simulink model "POINTING_2"  (R2022b)
settings: Solver=VariableStepAuto  StartTime=0.0  StopTime=36000  RelTol=1e-3
values from neighbouring files (symbols this model uses):
  A0 = angle2dcm(E1+0.7,E2+0.4,E3-1)    [Pointing_tuning.m]
  K_cz = sat.I/sat.I(3)*1e-4    [Pointing_tuning.m]    (also in fitnessfcn.m = X(4:6))
  K_w = 1e-2    (= 0.01)    [Pointing_tuning.m]    (also in fitnessfcn.m = X(7))
  n = sqrt(settings.mu/settings.a^3)    [Pointing_tuning.m]    (also in control_tuning.m)
undefined symbols (not defined in the file or in its folder): environment, r0, sat, settings, v0
libraries: matrix_library x7, vrlib x4, cstblocks x1
settings Model: Creator=brent  LastModifiedBy=brent

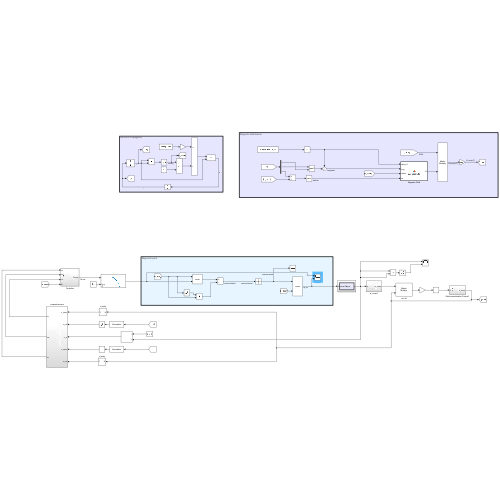
[thumbnail: Simulink's stored preview of the top-level diagram]
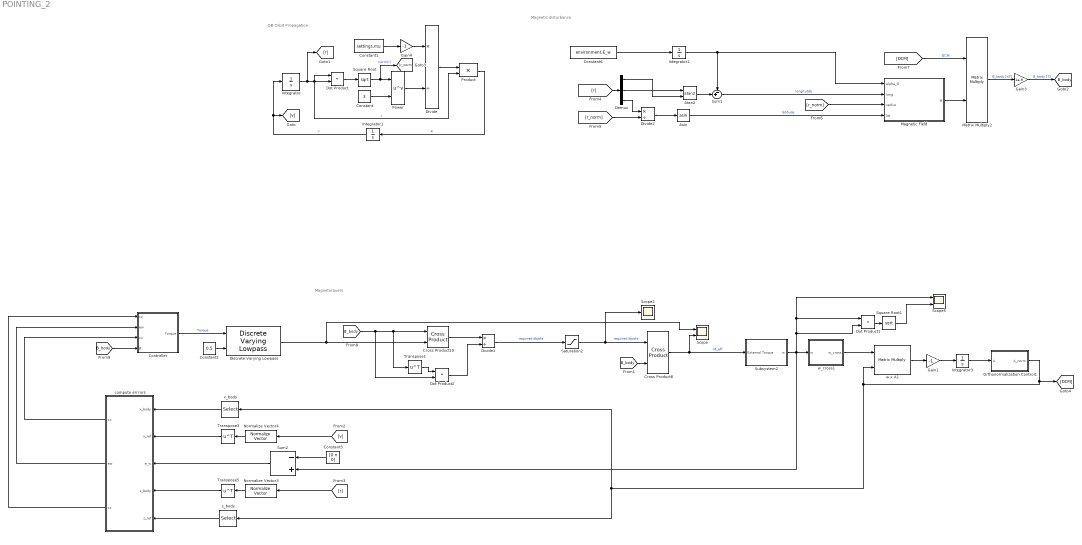
== system POINTING_2 ==
  note: Magnetic disturbance
  note: OB Orbit Propagation
  note: Magnetorquers
  " w x A1" : Product  Multiplication=Matrix(*)
  Asin : Trigonometry  Operator=asin
  Atan2 : Trigonometry  Operator=atan2
  Constant : Constant  Value=3
  Constant1 : Constant  Value=settings.mu
  Constant2 : Constant  Value=0.5
  Constant3 : Constant  Value=[0 n 0]
  Constant6 : Constant  Value=environment.E_w
  Controller : Subsystem
  Cross Product10 : matrix_library/Cross Product
  Cross Product8 : matrix_library/Cross Product
  Demux : Demux  Outputs=3
  Discrete Varying Lowpass : cstblocks/Linear Parameter Varying/Discrete Varying Lowpass  N=4  w0=0  Ts=1
  Divide : Product  Inputs=*/
  Divide1 : Product  Inputs=*/  RndMeth=Zero  SaturateOnIntegerOverflow=on
  Divide2 : Product  Inputs=*/
  Dot Product : DotProduct  OutDataTypeStr=Inherit: Inherit via internal rule
  Dot Product1 : DotProduct  OutDataTypeStr=Inherit: Inherit via internal rule
  Dot Product2 : DotProduct  OutDataTypeStr=Inherit: Inherit via internal rule
  Gain1 : Gain  Gain=-1
  Gain3 : Gain  Gain=1e-9
  Gain4 : Gain  Gain=-1
  Integrator : Integrator  InitialCondition=r0
  Integrator1 : Integrator  InitialCondition=v0
  Integrator2 : Integrator  InitialCondition=environment.theta_G0
  Integrator3 : Integrator  InitialCondition=A0
  Magnetic Field : MATLAB Function  TreatAsAtomicUnit=on
  Matrix Multiply2 : Product  Multiplication=Matrix(*)
  Normalize Vector3 : vrlib/Utilities/Normalize Vector  maxzero=0
  Normalize Vector4 : vrlib/Utilities/Normalize Vector  maxzero=0
  Orthonormalization Control1 : Subsystem
  Power : Math  Operator=pow
  Product : Product
  Saturation2 : Saturate  UpperLimit=120  LowerLimit=-120
  Scope : Scope  NumInputPorts=2
  Scope2 : Scope
  Scope5 : Scope  NumInputPorts=2
  Square Root : Sqrt
  Square Root1 : Sqrt
  Subsystem2 : Subsystem
  Sum1 : Sum  Inputs=-+|
  Sum2 : Sum  Inputs=-+
  Transpose1 : Math  Operator=transpose
  Transpose3 : Math  Operator=transpose
  Transpose5 : Math  Operator=transpose
  compute errrors : Subsystem
  w_cross1 : Subsystem
  x_body : Selector  NumberOfDimensions=2  InputPortWidth=3  IndexOptions=Index vector (dialog),Index vector (dialog)  Indices=[1],[1 2 3]  OutputSizes=1,1
  z_body : Selector  NumberOfDimensions=2  InputPortWidth=3  IndexOptions=Index vector (dialog),Index vector (dialog)  Indices=[3],[1 2 3]  OutputSizes=1,1
  tag scope: B_body=global
  wires:
  Divide2/1 -> Asin/1
  Constant6/1 -> Integrator2/1
  [DCM] -> Matrix Multiply2/1  "DCM"
  Demux/3 -> Divide2/1
  Matrix Multiply2/1 -> Gain3/1  "B_body [nT]"
  Demux/2 -> Atan2/1
  [r] -> Demux/1
  [r_norm] -> Magnetic Field/3(radius)
  Gain3/1 -> [B_body]  "B_body [T]"
  Demux/1 -> Atan2/2
  Integrator2/1 -> Sum1/1, Magnetic Field/1(alpha_G)
  Asin/1 -> Magnetic Field/4(lat)  "latitude"
  Atan2/1 -> Sum1/2
  Constant/1 -> Power/2
  Product/1 -> Integrator1/1  "a"
  Integrator/1 -> [r], Product/2, Dot Product/2, Dot Product/1  "r"
  Integrator1/1 -> [v], Integrator/1  "v"
  Dot Product/1 -> Square Root/1
  Magnetic Field/1(B) -> Matrix Multiply2/2
  Sum1/1 -> Magnetic Field/2(long)  "longitutde"
  Constant1/1 -> Gain4/1
  [r_norm] -> Divide2/2
  Power/1 -> Divide/2
  Gain4/1 -> Divide/1
  Square Root/1 -> [r_norm], Power/1  "norm(r)"
  Divide/1 -> Product/1
  Square Root1/1 -> Scope5/2
  Subsystem2/1(w) -> Sum2/2, w_cross1/1(w), Dot Product1/1, Scope5/1, Dot Product1/2
  Orthonormalization Control1/1(A_norm) -> [DCM], x_body/1, z_body/1, " w x A1"/2
  " w x A1"/1 -> Gain1/1
  w_cross1/1(w_cross) -> " w x A1"/1
  Integrator3/1 -> Orthonormalization Control1/1(A)
  Dot Product1/1 -> Square Root1/1
  Gain1/1 -> Integrator3/1
  [B_body] -> Transpose1/1, Cross Product10/1, Dot Product2/2
  Transpose1/1 -> Dot Product2/1
  Dot Product2/1 -> Divide1/2
  Cross Product10/1 -> Divide1/1
  Divide1/1 -> Saturation2/1  "required dipole"
  [B_body] -> Cross Product8/2
  Cross Product8/1 -> Scope/2, Subsystem2/1(External Torque)  "M_eff"
  Saturation2/1 -> Cross Product8/1, Scope2/1  "required dipole"
  Controller/1(Torque) -> Discrete Varying Lowpass/1  "Torque"
  Constant3/1 -> Sum2/1
  Discrete Varying Lowpass/1 -> Scope/1, Cross Product10/2
  Constant2/1 -> Discrete Varying Lowpass/2
  Normalize Vector4/1 -> Transpose3/1
  [r] -> Normalize Vector3/1
  [v] -> Normalize Vector4/1
  Normalize Vector3/1 -> Transpose5/1
  x_body/1 -> compute errrors/1(x_body)
  Transpose3/1 -> compute errrors/2(x_ref)
  Sum2/1 -> compute errrors/3(e_w)
  Transpose5/1 -> compute errrors/4(z_body)
  z_body/1 -> compute errrors/5(z_ref)
  compute errrors/1(cx) -> Controller/3(cx)
  compute errrors/2(ew) -> Controller/2(ew)
  compute errrors/3(cz) -> Controller/1(cz)
  [B_body] -> Controller/4(B)

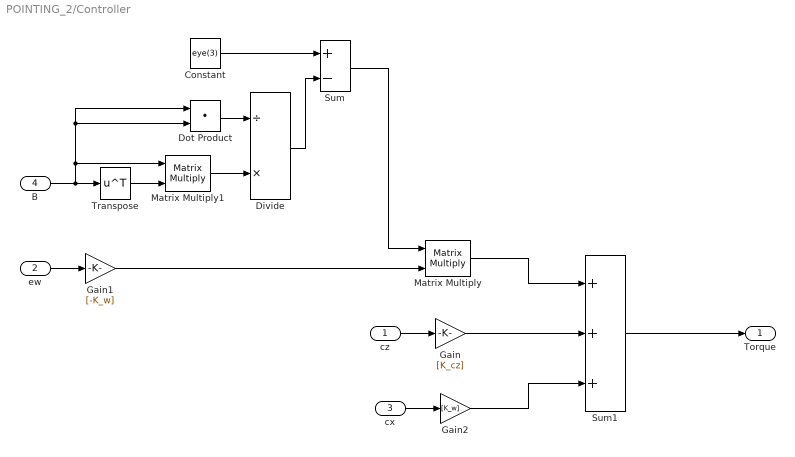
== system POINTING_2/Controller ==
  cz : Inport
  ew : Inport  Port=2
  cx : Inport  Port=3
  B : Inport  Port=4
  Constant : Constant  Value=eye(3)
  Divide : Product  Inputs=/*
  Dot Product : DotProduct  OutDataTypeStr=Inherit: Inherit via internal rule
  Gain : Gain  Gain=[K_cz]
  Gain1 : Gain  Gain=[-K_w]
  Gain2 : Gain  Gain=[K_w]
  Matrix Multiply : Product  Multiplication=Matrix(*)
  Matrix Multiply1 : Product  Multiplication=Matrix(*)
  Sum : Sum  Inputs=+-
  Sum1 : Sum  Inputs=+++
  Transpose : Math  Operator=transpose
  Torque : Outport
  wires:
  cz/1 -> Gain/1
  ew/1 -> Gain1/1
  cx/1 -> Gain2/1
  Gain1/1 -> Matrix Multiply/2
  Constant/1 -> Sum/1
  B/1 -> Dot Product/2, Dot Product/1, Matrix Multiply1/1, Transpose/1
  Transpose/1 -> Matrix Multiply1/2
  Matrix Multiply1/1 -> Divide/2
  Dot Product/1 -> Divide/1
  Divide/1 -> Sum/2
  Sum/1 -> Matrix Multiply/1
  Gain/1 -> Sum1/2
  Matrix Multiply/1 -> Sum1/1
  Gain2/1 -> Sum1/3
  Sum1/1 -> Torque/1

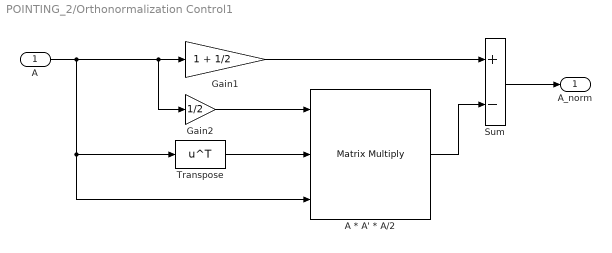
== system POINTING_2/Orthonormalization Control1 ==
  A : Inport
  " A * A' * A/2" : Product  Inputs=3  Multiplication=Matrix(*)
  Gain1 : Gain  Gain=1 + 1/2
  Gain2 : Gain  Gain=1/2
  Sum : Sum  Inputs=+-
  Transpose : Math  Operator=transpose
  A_norm : Outport
  wires:
  A/1 -> Transpose/1, " A * A' * A/2"/3, Gain1/1, Gain2/1
  Gain1/1 -> Sum/1
  " A * A' * A/2"/1 -> Sum/2
  Sum/1 -> A_norm/1
  Gain2/1 -> " A * A' * A/2"/1
  Transpose/1 -> " A * A' * A/2"/2

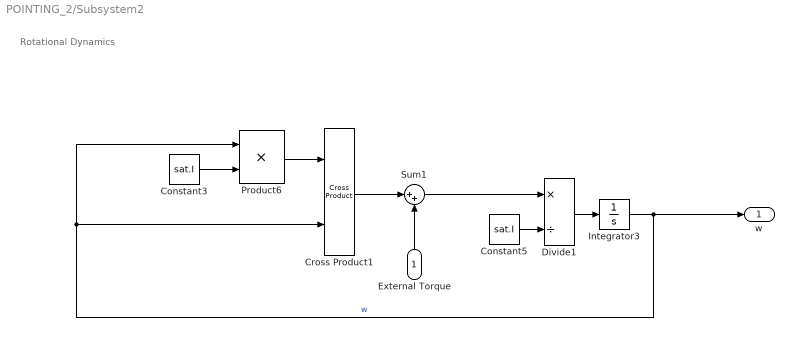
== system POINTING_2/Subsystem2 ==
  note: Rotational Dynamics
  External Torque : Inport
  Constant3 : Constant  Value=sat.I
  Constant5 : Constant  Value=sat.I
  Cross Product1 : matrix_library/Cross Product
  Divide1 : Product  Inputs=*/
  Integrator3 : Integrator  InitialCondition=settings.w0
  Product6 : Product
  Sum1 : Sum  Inputs=|++
  w : Outport
  wires:
  Constant5/1 -> Divide1/2
  Sum1/1 -> Divide1/1
  External Torque/1 -> Sum1/2
  Integrator3/1 -> w/1, Cross Product1/2, Product6/1  "w"
  Divide1/1 -> Integrator3/1
  Cross Product1/1 -> Sum1/1
  Constant3/1 -> Product6/2
  Product6/1 -> Cross Product1/1

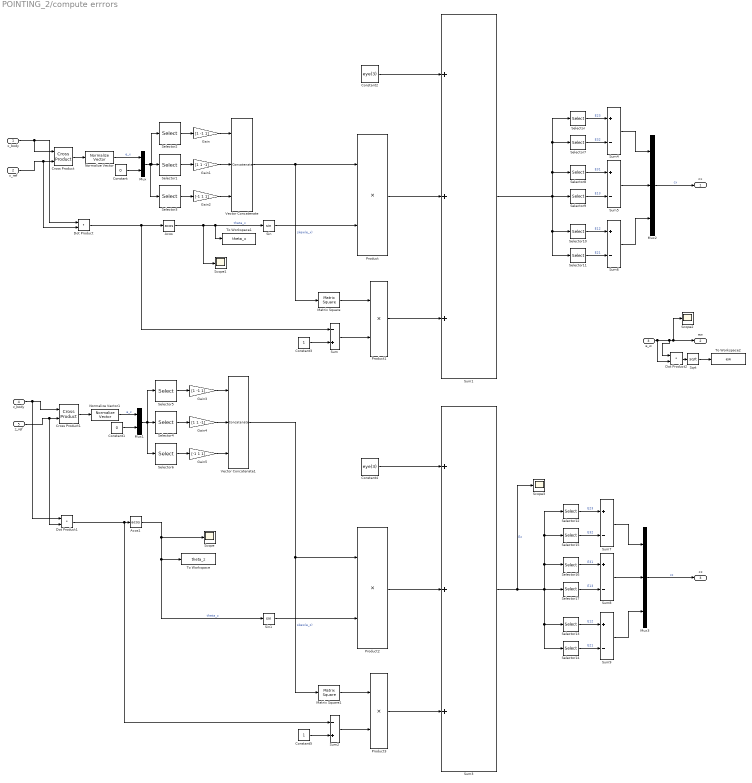
== system POINTING_2/compute errrors ==
  x_body : Inport
  x_ref : Inport  Port=2
  e_w : Inport  Port=3
  z_body : Inport  Port=4
  z_ref : Inport  Port=5
  Acos : Trigonometry  Operator=acos
  Acos1 : Trigonometry  Operator=acos
  Constant : Constant  Value=0
  Constant1 : Constant  Value=0
  Constant2 : Constant  Value=eye(3)
  Constant3 : Constant
  Constant4 : Constant  Value=eye(3)
  Constant5 : Constant
  Cross Product : matrix_library/Cross Product
  Cross Product1 : matrix_library/Cross Product
  Dot Product : DotProduct  OutDataTypeStr=Inherit: Inherit via internal rule
  Dot Product1 : DotProduct  OutDataTypeStr=Inherit: Inherit via internal rule
  Dot Product2 : DotProduct  OutDataTypeStr=Inherit: Inherit via internal rule
  Gain : Gain  Gain=[1 -1 1]
  Gain1 : Gain  Gain=[1 1 -1]
  Gain2 : Gain  Gain=[-1 1 1]
  Gain3 : Gain  Gain=[1 -1 1]
  Gain4 : Gain  Gain=[1 1 -1]
  Gain5 : Gain  Gain=[-1 1 1]
  Matrix Square : matrix_library/Matrix Square  OutMin=[]  OutMax=[]
      settings: LibrarySourceBlock=|
      | simulink/Matrix
      | Operations/Matrix
      | Square
  Matrix Square1 : matrix_library/Matrix Square  OutMin=[]  OutMax=[]
      settings: LibrarySourceBlock=|
      | simulink/Matrix
      | Operations/Matrix
      | Square
  Mux : Mux  Inputs=2
  Mux1 : Mux  Inputs=2
  Mux2 : Mux  Inputs=3
  Mux3 : Mux  Inputs=3
  Normalize Vector : vrlib/Utilities/Normalize Vector  maxzero=0
  Normalize Vector1 : vrlib/Utilities/Normalize Vector  maxzero=0
  Product{,1..3} (4 alike) : Product
  Scope{,1..3} (4 alike) : Scope
  Selector : Selector  NumberOfDimensions=2  InputPortWidth=3  IndexOptions=Index vector (dialog),Index vector (dialog)  Indices=[2],3  OutputSizes=1,1
  Selector1 : Selector  InputPortWidth=4  IndexOptions=Index vector (dialog)  Indices=[3 4 1]  OutputSizes=1
  Selector10 : Selector  NumberOfDimensions=2  InputPortWidth=3  IndexOptions=Index vector (dialog),Index vector (dialog)  Indices=1,2  OutputSizes=1,1
  Selector11 : Selector  NumberOfDimensions=2  InputPortWidth=3  IndexOptions=Index vector (dialog),Index vector (dialog)  Indices=2,1  OutputSizes=1,1
  Selector12 : Selector  NumberOfDimensions=2  InputPortWidth=3  IndexOptions=Index vector (dialog),Index vector (dialog)  Indices=[2],3  OutputSizes=1,1
  Selector13 : Selector  NumberOfDimensions=2  InputPortWidth=3  IndexOptions=Index vector (dialog),Index vector (dialog)  Indices=1,2  OutputSizes=1,1
  Selector14 : Selector  NumberOfDimensions=2  InputPortWidth=3  IndexOptions=Index vector (dialog),Index vector (dialog)  Indices=2,1  OutputSizes=1,1
  Selector15 : Selector  NumberOfDimensions=2  InputPortWidth=3  IndexOptions=Index vector (dialog),Index vector (dialog)  Indices=3,2  OutputSizes=1,1
  Selector16 : Selector  NumberOfDimensions=2  InputPortWidth=3  IndexOptions=Index vector (dialog),Index vector (dialog)  Indices=3,1  OutputSizes=1,1
  Selector17 : Selector  NumberOfDimensions=2  InputPortWidth=3  IndexOptions=Index vector (dialog),Index vector (dialog)  Indices=1,3  OutputSizes=1,1
  Selector2 : Selector  InputPortWidth=4  IndexOptions=Index vector (dialog)  Indices=[4 3 2]  OutputSizes=1
  Selector3 : Selector  InputPortWidth=4  IndexOptions=Index vector (dialog)  Indices=[2 1 4]  OutputSizes=1
  Selector4 : Selector  InputPortWidth=4  IndexOptions=Index vector (dialog)  Indices=[3 4 1]  OutputSizes=1
  Selector5 : Selector  InputPortWidth=4  IndexOptions=Index vector (dialog)  Indices=[4 3 2]  OutputSizes=1
  Selector6 : Selector  InputPortWidth=4  IndexOptions=Index vector (dialog)  Indices=[2 1 4]  OutputSizes=1
  Selector7 : Selector  NumberOfDimensions=2  InputPortWidth=3  IndexOptions=Index vector (dialog),Index vector (dialog)  Indices=3,2  OutputSizes=1,1
  Selector8 : Selector  NumberOfDimensions=2  InputPortWidth=3  IndexOptions=Index vector (dialog),Index vector (dialog)  Indices=3,1  OutputSizes=1,1
  Selector9 : Selector  NumberOfDimensions=2  InputPortWidth=3  IndexOptions=Index vector (dialog),Index vector (dialog)  Indices=1,3  OutputSizes=1,1
  Sin : Trigonometry
  Sin1 : Trigonometry
  Sqrt : Sqrt
  Sum : Sum  Inputs=-+
  Sum1 : Sum  Inputs=+++
  Sum2 : Sum  Inputs=-+
  Sum3 : Sum  Inputs=+++
  Sum{4..9} (6 alike) : Sum  Inputs=+-
  To Workspace : ToWorkspace  VariableName=theta_z  SampleTime=-1
  To Workspace1 : ToWorkspace  VariableName=theta_x  SampleTime=-1
  To Workspace2 : ToWorkspace  VariableName=ew  SampleTime=-1
  Vector Concatenate : Concatenate  NumInputs=3  Mode=Multidimensional array
  Vector Concatenate1 : Concatenate  NumInputs=3  Mode=Multidimensional array
  cx : Outport
  ew : Outport  Port=2
  cz : Outport  Port=3
  wires:
  x_body/1 -> Dot Product/1, Cross Product/1
  x_ref/1 -> Dot Product/2, Cross Product/2
  Cross Product/1 -> Normalize Vector/1
  Cross Product1/1 -> Normalize Vector1/1
  Normalize Vector/1 -> Mux/1  "e_x"
  Normalize Vector1/1 -> Mux1/1  "e_z"
  Constant/1 -> Mux/2
  Mux/1 -> Selector3/1, Selector1/1, Selector2/1
  Selector2/1 -> Gain/1
  Selector1/1 -> Gain1/1
  Selector3/1 -> Gain2/1
  Gain1/1 -> Vector Concatenate/2
  Gain2/1 -> Vector Concatenate/3
  Gain/1 -> Vector Concatenate/1
  Gain3/1 -> Vector Concatenate1/1
  Gain5/1 -> Vector Concatenate1/3
  Gain4/1 -> Vector Concatenate1/2
  Selector6/1 -> Gain5/1
  Selector4/1 -> Gain4/1
  Selector5/1 -> Gain3/1
  Mux1/1 -> Selector5/1, Selector4/1, Selector6/1
  Constant1/1 -> Mux1/2
  Vector Concatenate1/1 -> Matrix Square1/1, Product2/1  "skew(e_z)"
  Dot Product1/1 -> Sum2/1, Acos1/1
  z_ref/1 -> Dot Product1/2, Cross Product1/2
  z_body/1 -> Dot Product1/1, Cross Product1/1
  Acos/1 -> Scope1/1, To Workspace1/1, Sin/1  "theta_x"
  Acos1/1 -> Scope/1, Sin1/1, To Workspace/1  "theta_z"
  Constant3/1 -> Sum/2
  Dot Product/1 -> Acos/1, Sum/1
  Vector Concatenate/1 -> Product/1, Matrix Square/1  "skew(e_x)"
  Sin/1 -> Product/2
  Matrix Square/1 -> Product1/1
  Sum/1 -> Product1/2
  Constant2/1 -> Sum1/1
  Product/1 -> Sum1/2
  Product1/1 -> Sum1/3
  Sum1/1 -> Selector9/1, Selector8/1, Selector7/1, Selector/1, Selector10/1, Selector11/1
  Sum3/1 -> Scope3/1, Selector14/1, Selector13/1, Selector12/1, Selector15/1, Selector16/1, Selector17/1  "Ez"
  Product3/1 -> Sum3/3
  Product2/1 -> Sum3/2
  Constant4/1 -> Sum3/1
  Sum2/1 -> Product3/2
  Matrix Square1/1 -> Product3/1
  Sin1/1 -> Product2/2
  Constant5/1 -> Sum2/2
  Selector/1 -> Sum4/1  "E23"
  Selector7/1 -> Sum4/2  "E32"
  Selector8/1 -> Sum5/1  "E31"
  Selector9/1 -> Sum5/2  "E13"
  Selector10/1 -> Sum6/1  "E12"
  Selector11/1 -> Sum6/2  "E21"
  Sum5/1 -> Mux2/2
  Sum4/1 -> Mux2/1
  Sum6/1 -> Mux2/3
  Mux2/1 -> cx/1  "cx"
  Mux3/1 -> cz/1  "cz"
  Sum9/1 -> Mux3/3
  Sum7/1 -> Mux3/1
  Sum8/1 -> Mux3/2
  Selector14/1 -> Sum9/2  "E21"
  Selector13/1 -> Sum9/1  "E12"
  Selector17/1 -> Sum8/2  "E13"
  Selector16/1 -> Sum8/1  "E31"
  Selector15/1 -> Sum7/2  "E32"
  Selector12/1 -> Sum7/1  "E23"
  Sqrt/1 -> To Workspace2/1
  e_w/1 -> Dot Product2/2, Dot Product2/1, Scope2/1, ew/1
  Dot Product2/1 -> Sqrt/1

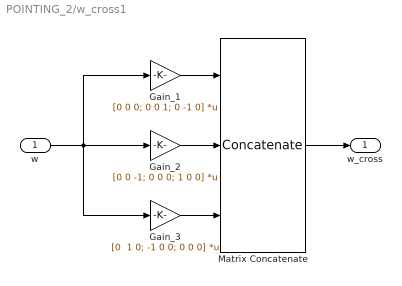
== system POINTING_2/w_cross1 ==
  w : Inport
  Gain_1 : Gain  Gain=[0 0 0; 0 0 1; 0 -1 0]  Multiplication=Matrix(K*u)
  Gain_2 : Gain  Gain=[0 0 -1; 0 0 0; 1 0 0]  Multiplication=Matrix(K*u)
  Gain_3 : Gain  Gain="[0  1 0; -1 0 0; 0 0 0]"  Multiplication=Matrix(K*u)
  Matrix Concatenate : Concatenate  NumInputs=3  Mode=Multidimensional array  ConcatenateDimension=2
  w_cross : Outport
  wires:
  w/1 -> Gain_2/1, Gain_1/1, Gain_3/1
  Gain_3/1 -> Matrix Concatenate/3
  Gain_2/1 -> Matrix Concatenate/2
  Gain_1/1 -> Matrix Concatenate/1
  Matrix Concatenate/1 -> w_cross/1

== matlab function POINTING_2/Magnetic Field ==
  data: alpha_G input; long input; radius input; B output; lat input; environment parameter; settings parameter
function B = magneticField(alpha_G,long,radius,lat,environment,settings)
%{  
    Return the magnetic field component in inertial reference frame

%}
theta = (pi/2-lat);     % theta is the colatitude [rad]
alpha = long + alpha_G; 

g = environment.WMM.g;
h = environment.WMM.h;
K = environment.WMM.K;
R = environment.R;
N = settings.N;

%% P-dP
% validated through the P and dP tables in "Jeremy Davis, Mathematical Modeling of Earthas Magnetic
% Field, 2004"

%%%%%%%%%%%%%%%%%%%%%%%%%%%%%%%%%%%%%%%%%%%%%%%%%%%%%%%%%%%%%%%%%%%%%%%%%%%%%%%%%%%%%%%%%%%%%%%%
% P_{(n),(m+1)}: 
% given P(a,b) -> n=a, m=b-1
% n from 1 to N
% m from 0 to N
% N order of accuracy
%%%%%%%%%%%%%%%%%%%%%%%%%%%%%%%%%%%%%%%%%%%%%%%%%%%%%%%%%%%%%%%%%%%%%%%%%%%%%%%%%%%%%%%%%%%%%%%%

P = zeros(N,N+1);
dP = zeros(N,N+1);

P_00 = 1;
dP_00 = 0;

P_01 = 0; 
dP_01 = 0;

P(1,1) = cos(theta); % n=1, m=0
dP(1,1) = -sin(theta)*P_00; 

P(1,2) = sin(theta);  % n=1, m=1
dP(1,2) = cos(theta)*P_00;

for i = 2:N % ciclo in n a partire da n=2 a n=N
    for j = 0:i % ciclo in m da m=0 a m=n
        if j == i
        P(i,j+1) = sin(theta)*P(i-1,j);
        dP(i,j+1) = sin(theta)*dP(i-1,j) + cos(theta)*P(i-1,j);
        elseif i < 3
            if j == 0 % n=2, m=0
            P(i,j+1) = cos(theta)*P(i-1,j+1) - K(i,j+1)*P_00;
            dP(i,j+1) = -sin(theta)*P(i-1,j+1) + cos(theta)*dP(i-1,j+1) ...
                - K(i,j+1)*dP_00;
            elseif j == 1 % n=2, m=1
                P(i,j+1) = cos(theta)*P(i-1,j+1) - K(i,j+1)*P_01;
                dP(i,j+1) = -sin(theta)*P(i-1,j+1) + cos(theta)*dP(i-1,j+1)...
                    - K(i,j+1)*dP_01;
            end
        else
            P(i,j+1) = cos(theta)*P(i-1,j+1) - K(i,j+1)*P(i-2,j+1);
            dP(i,j+1) = -sin(theta)*P(i-1,j+1) + cos(theta)*dP(i-1,j+1) ...
                - K(i,j+1)*dP(i-2,j+1);
        end
    end
end

%% Magnetic Field

B_r = 0;
B_th = 0;
B_phi = 0;

%indice i scorre n da 1 a N
%indice j scorre m da 0 a n

for m = 0:N
    for n = 1:N
        if m<=n
            B_r = B_r + (R/radius)^(n+2)*(n+1)*...
                ((g(n,m+1)*cos(m*long) + h(n,m+1)*sin(m*long))*P(n, m+1));
            B_th = B_th + (R/radius)^(n+2)*...
                ((g(n,m+1)*cos(m*long) + h(n,m+1)*sin(m*long))*dP(n, m+1));
            B_phi = B_phi + (R/radius)^(n+2)*...
                (m*(-g(n,m+1)*sin(m*long) + h(n,m+1)*cos(m*long))* P(n, m+1));

        end

    end
end

B_th = -B_th;
B_phi = -B_phi/sin(theta);

B_x = ( B_r*cos(lat) + B_th*sin(lat) ) * cos(alpha) - B_phi*sin(alpha);
B_y = ( B_r*cos(lat) + B_th*sin(lat) ) * sin(alpha) + B_phi*cos(alpha);
B_z = B_r*sin(lat) + B_th*cos(lat);

B = [B_x B_y B_z]';
